simulink subsystem "Encoder2D"  (R2024a)
settings: Solver=VariableStepAuto  StartTime=0.0  StopTime=10.0  RelTol=1e-3
undefined symbols (not defined in the file or in its folder): CPR, DiscIntNeverNeededParam, wheelBase, wheelRadius
settings Model: Creator=Peter  LastModifiedBy=Peter

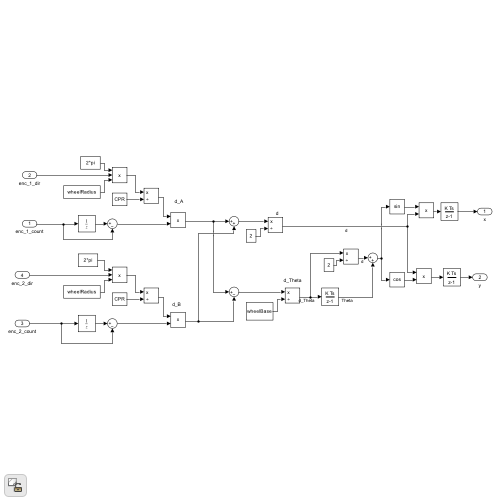
[thumbnail: Simulink's stored preview of the top-level diagram]
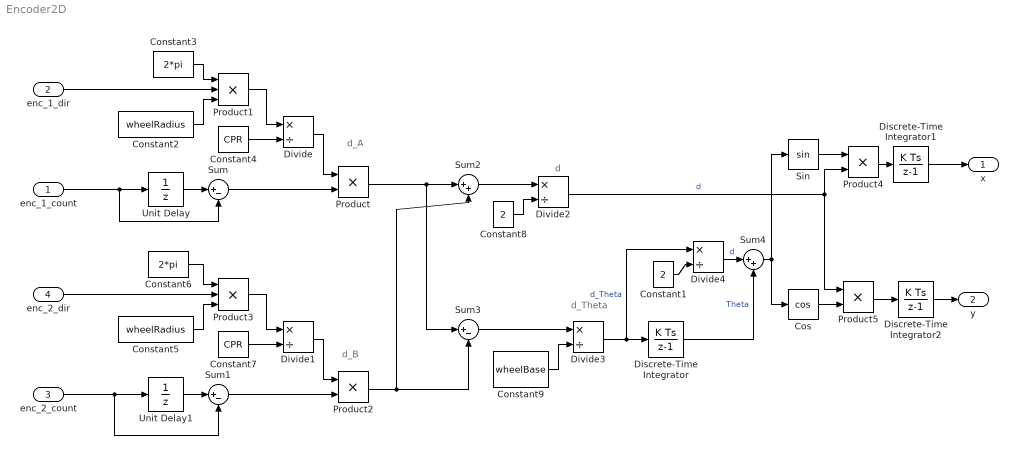
== system Encoder2D ==
  note: d_Theta
  note: d
  note: d_A
  note: d_B
  enc_1_count : Inport
  enc_1_dir : Inport  Port=2
  enc_2_count : Inport  Port=3
  enc_2_dir : Inport  Port=4
  Constant1 : Constant  Value=2
  Constant2 : Constant  Value=wheelRadius
  Constant3 : Constant  Value=2*pi
  Constant4 : Constant  Value=CPR
  Constant5 : Constant  Value=wheelRadius
  Constant6 : Constant  Value=2*pi
  Constant7 : Constant  Value=CPR
  Constant8 : Constant  Value=2
  Constant9 : Constant  Value=wheelBase
  Cos : Trigonometry  Operator=cos
  Discrete-Time Integrator : DiscreteIntegrator  SampleTime=-1  ICPrevOutput=DiscIntNeverNeededParam  ICPrevScaledInput=DiscIntNeverNeededParam
  Discrete-Time Integrator1 : DiscreteIntegrator  SampleTime=-1  ICPrevOutput=DiscIntNeverNeededParam  ICPrevScaledInput=DiscIntNeverNeededParam
  Discrete-Time Integrator2 : DiscreteIntegrator  SampleTime=-1  ICPrevOutput=DiscIntNeverNeededParam  ICPrevScaledInput=DiscIntNeverNeededParam
  Divide{,1..4} (5 alike) : Product  Inputs=*/
  Product{,2,4..5} (4 alike) : Product
  Product1 : Product  Inputs=3
  Product3 : Product  Inputs=3
  Sin : Trigonometry
  Sum : Sum  Inputs=|+-
  Sum1 : Sum  Inputs=|+-
  Sum2 : Sum  Inputs=|++
  Sum3 : Sum  Inputs=|+-
  Sum4 : Sum  Inputs=|++
  Unit Delay : UnitDelay  SampleTime=-1  HasFrameUpgradeWarning=on
  Unit Delay1 : UnitDelay  SampleTime=-1  HasFrameUpgradeWarning=on
  x : Outport  OutDataTypeStr=single
  y : Outport  Port=2  OutDataTypeStr=single
  wires:
  Discrete-Time Integrator1/1 -> x/1
  Discrete-Time Integrator2/1 -> y/1
  enc_1_count/1 -> Unit Delay/1, Sum/2
  Unit Delay/1 -> Sum/1
  Sum/1 -> Product/2
  enc_1_dir/1 -> Product1/2
  Constant2/1 -> Product1/3
  Constant3/1 -> Product1/1
  Product1/1 -> Divide/1
  Constant4/1 -> Divide/2
  Divide/1 -> Product/1
  enc_2_count/1 -> Unit Delay1/1, Sum1/2
  Sum1/1 -> Product2/2
  Constant6/1 -> Product3/1
  Constant7/1 -> Divide1/2
  Product3/1 -> Divide1/1
  Constant5/1 -> Product3/3
  Divide1/1 -> Product2/1
  enc_2_dir/1 -> Product3/2
  Unit Delay1/1 -> Sum1/1
  Product/1 -> Sum2/1, Sum3/1
  Product2/1 -> Sum2/2, Sum3/2
  Sum2/1 -> Divide2/1
  Constant8/1 -> Divide2/2
  Sum3/1 -> Divide3/1
  Constant9/1 -> Divide3/2
  Divide3/1 -> Discrete-Time Integrator/1, Divide4/1  "d_Theta"
  Discrete-Time Integrator/1 -> Sum4/2  "Theta"
  Divide2/1 -> Product5/1, Product4/2  "d"
  Constant1/1 -> Divide4/2
  Divide4/1 -> Sum4/1  "d"
  Sum4/1 -> Sin/1, Cos/1
  Sin/1 -> Product4/1
  Cos/1 -> Product5/2
  Product5/1 -> Discrete-Time Integrator2/1
  Product4/1 -> Discrete-Time Integrator1/1
